simulink model "Model1"  (R2018a)
settings: Solver=VariableStepAuto  StartTime=0.0  StopTime=10.0  RelTol=1e-3
values from neighbouring files (symbols this model uses):
  x0 = [pi,0,0.1,0,0]'    [7_8.m]    (also in CEEProject.m = [0.1,0,0,0,0]'; CEEproject.m = [0.1,0,0,0,0]'; Ines.m = [pi,0,0.4,0,0]'; MCsynthesis.m = [pi/2,0,0.18,0,0]')
undefined symbols (not defined in the file or in its folder): A, B, K
settings Model: Creator=miguelsilva  LastModifiedBy=leonardopedroso
settings DebuggingCC: LibraryContextMissingDiagnostic=warning
settings SFSimCC: SimUseLocalCustomCode=on
settings RTWCC: RTWUseLocalCustomCode=on

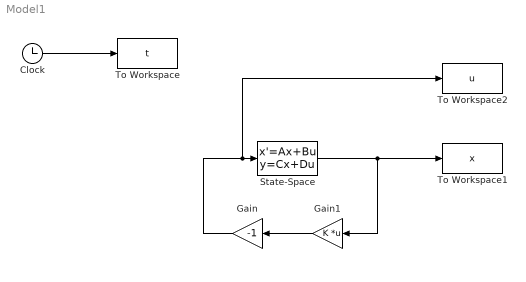
== system Model1 ==
  Clock : Clock
  Gain : Gain  Gain=-1
  Gain1 : Gain  Gain=K  Multiplication=Matrix(K*u)
  State-Space : StateSpace  A=A  B=B  C=eye(5)  D=zeros(5,1)  InitialCondition=x0  ContinuousStateAttributes={'x1','x2','x3','x4','x5'}
  To Workspace : ToWorkspace  VariableName=t  SampleTime=-1
  To Workspace1 : ToWorkspace  VariableName=x  SampleTime=-1
  To Workspace2 : ToWorkspace  VariableName=u  SampleTime=-1
  wires:
  State-Space/1 -> Gain1/1, To Workspace1/1
  Gain1/1 -> Gain/1
  Gain/1 -> To Workspace2/1, State-Space/1
  Clock/1 -> To Workspace/1
